simulink model "autosar"  (R2021a)
settings: Solver=FixedStepDiscrete  StartTime=0.0  StopTime=10.0  RelTol=1e-3  EnableMultiTasking=on
libraries: autosarlibdem x1, autosarspkglib_internal x1
settings Model: Creator=Aly  LastModifiedBy=Aly
settings SolverCC: AlgebraicLoopSolver=TrustRegion  AutoInsertRateTranBlk=on  InsertRTBMode=Never (minimum delay)
settings OptimizationCC: DefaultParameterBehavior=Inlined  EnhancedBackFolding=on  PassReuseOutputArgsAs=Individual arguments  ZeroExternalMemoryAtStartup=off  ZeroInternalMemoryAtStartup=off  OptimizeBlockOrder=speed  DifferentSizesBufferReuse=on  OptimizationCustomize=off  EfficientTunableParamExpr=on
settings DebuggingCC: MultiTaskDSMMsg=none  MultiTaskRateTransMsg=warning  ParameterTunabilityLossMsg=error  UnconnectedInputMsg=none  UnconnectedOutputMsg=none  SFMachineParentedDataDiag=warning
settings SFSimCC: MATLABDynamicMemAlloc=off
settings RTWCC: Description=AUTOSAR  SystemTargetFile=autosar.tlc  GenCodeOnly=on  TemplateMakefile=ert_default_tmf  IncludeHyperlinkInReport=on
settings CodeAppCC: ForceParamTrailComments=on  IgnoreCustomStorageClasses=off  OperatorAnnotations=on  SimulinkDataObjDesc=on  SFDataObjDesc=on  InsertBlockDesc=on
settings STFCustomTargetCC: TargetLangStandard=C99 (ISO)  MultiwordLength=256  ParMdlRefBuildCompliant=on  CompOptLevelCompliant=on  IncludeMdlTerminateFcn=off  CombineOutputUpdateFcns=on  SuppressErrorStatus=on  ERTCustomFileBanners=on  SupportNonFinite=off  SupportComplex=off  SupportContinuousTime=off  SupportNonInlinedSFcns=off  RemoveResetFunc=on  MATLABClassNameForMDSCustomization=Simulink.SoftwareTarget.ERTCustomization  AutosarCompliant=on  GRTInterface=off  LookupTableObjectStructAxisOrder=2,1,3,4,...  LUTObjectStructOrderEvenSpacing=Size,Table,Breakpoints  SystemTargetFile=autosar.tlc
settings ERTTargetCC: TargetLangStandard=C99 (ISO)  ConcurrentExecutionCompliant=off  IncludeMdlTerminateFcn=off  SuppressErrorStatus=on  SupportNonFinite=off  SupportComplex=off  ModelStepFunctionPrototypeControlCompliant=off  CPPClassGenCompliant=off  AutosarCompliant=on  LookupTableObjectStructAxisOrder=2,1,3,4,...  LUTObjectStructOrderEvenSpacing=Size,Table,Breakpoints  InlinedParameterPlacement=NonHierarchical  ERTCustomFileTemplate=example_file_process.tlc

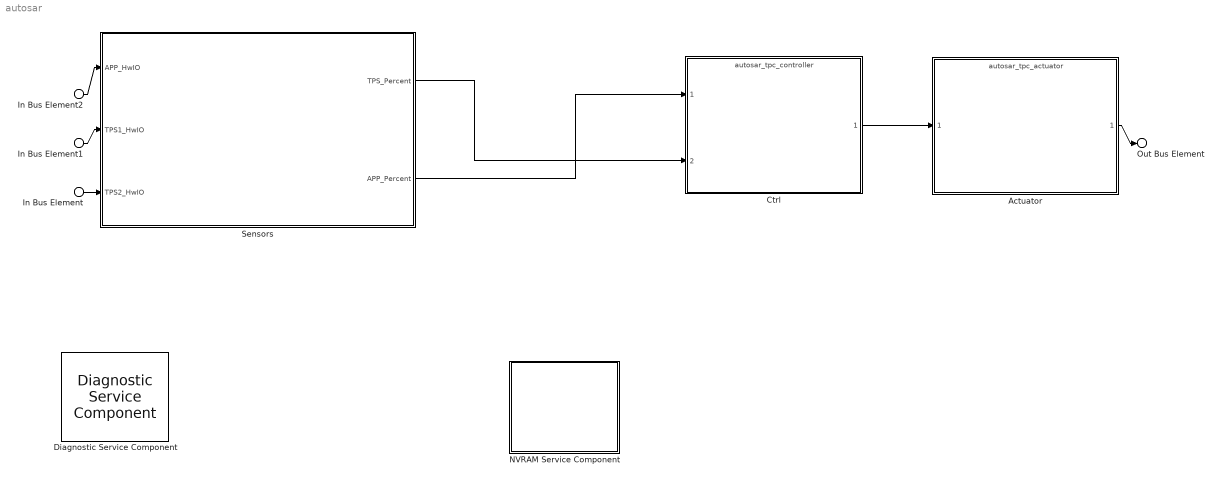
== system autosar ==
  In Bus Element2 : Inport  PortName=APP_HwIO
  In Bus Element1 : Inport  Port=2  PortName=TPS2_HwIO1
  In Bus Element : Inport  Port=3  PortName=TPS1_HwIO
  Actuator : ModelReference  ModelNameDialog=autosar_tpc_actuator  SimulationMode=Normal  ScheduleRates=on  ScheduleRatesWith=Schedule Editor  CodeInterface=Top model  ModelReferenceVersion=3.0
      settings: PortSchema="{\"entries\":[{\"content\":{\"headerSize\":38,\"margin\":15,\"minimumSpacing\":25,\"sides\":[{\"content\":{\"connectorIds\":[\"In1\"]},\"type\":\"ConnectorPlacement.EquallySpacedRectSide\",\"uuid\":\"26fd7ed6-1773-482a-a7b4-c0bab0c01c6e\"},{\"content\":{\"connectorIds\":[\"Out1\"],\"side\":\"RIGHT\"},\"type\":\"ConnectorPlacement.EquallySpacedRectSide\",\"uuid\":\"76751916-8837-4aff-8479-b4617ededb25\"},{\"content\":{\"connectorIds\":[],\"side\":\"TOP\"},\"type\":\"ConnectorPlacement.EquallySpacedRectSide\",\"uuid\":\"b9915de3-15c1-4354-81f8-a4ac649be3ef\"}]},\"type\":\"ConnectorPlacement.EquallySpacedConnector\",\"uuid\":\"5d928bdd-7cbf-4ffd-a89b-6f4194195412\"}],\"packageUris\":[\"http://schema.mathworks.com/mf0/Connector/19700101\"],\"version\":\"1.0\"}"
  Ctrl : ModelReference  ModelNameDialog=autosar_tpc_controller.slx  SimulationMode=Normal  ScheduleRates=on  ScheduleRatesWith=Schedule Editor  ModelReferenceVersion=3.0
      settings: PortSchema="{\"entries\":[{\"content\":{\"headerSize\":38,\"margin\":15,\"minimumSpacing\":25,\"sides\":[{\"content\":{\"connectorIds\":[\"In1\",\"In2\"]},\"type\":\"ConnectorPlacement.EquallySpacedRectSide\",\"uuid\":\"26fd7ed6-1773-482a-a7b4-c0bab0c01c6e\"},{\"content\":{\"connectorIds\":[\"Out1\"],\"side\":\"RIGHT\"},\"type\":\"ConnectorPlacement.EquallySpacedRectSide\",\"uuid\":\"76751916-8837-4aff-8479-b4617ededb25\"},{\"content\":{\"connectorIds\":[],\"side\":\"TOP\"},\"type\":\"ConnectorPlacement.EquallySpacedRectSide\",\"uuid\":\"b9915de3-15c1-4354-81f8-a4ac649be3ef\"}]},\"type\":\"ConnectorPlacement.EquallySpacedConnector\",\"uuid\":\"5d928bdd-7cbf-4ffd-a89b-6f4194195412\"}],\"packageUris\":[\"http://schema.mathworks.com/mf0/Connector/19700101\"],\"version\":\"1.0\"}"
  Diagnostic Service Component : autosarlibdem/Diagnostic Service Component  ClientPortNames={'S1StuckHigh', 'S1StuckLow', 'S2StuckHigh', 'S2StuckLow', 'TPS', 'TPS1StuckHigh', 'TPS1StuckLow', 'TPS2StuckHigh', 'TPS2StuckLow'}  ClientPortPortDefinedArguments={'1', '2', '3', '4', '5', '1', '2', '3', '4'}  MaxEventId=10  MaxFID=10  DemDebounceCounterIncrementStepSize=1  DemDebounceCounterDecrementStepSize=1  DemDebounceCounterFailedThreshold=2  DemDebounceCounterPassedThreshold=-1  InhibitionMatrix=[0 0 0 0 0 0 0 0 0 0 0;0 0 0 0 0 0 0 0 0 0 0;0 0 0 0 0 0 0 0 0 0 0;0 0 0 0 0 0 0 0 0 0 0;0 0 0 0 0 0 0 0 0 0 0;0 0 0 0 0 0 0 0 0 0 0;0 0 0 0 0 0 0 0 0 0 0;0 0 0 0 0 0 0 0 0 0 0;0 0 0 0 0 0 0 0 0 0 0;0 0 0 0 0 0 0 0 0 0 0;0 0 0 0 0 0 0 0 0 0 0]  EnableConditionIndexes=zeros(257,'uint8')  StorageConditionIndexes=zeros(257,'uint8')
      settings: SourceProductBaseCode=AS
  NVRAM Service Component : Subsystem  DialogController=bsw_create_dialog  mask(NVRAM Service Component){ClientPortNames={'S1LowSetPoint', 'S2LowSetPoint'}, ClientPortPortDefinedArguments={'1', '2'}, MaxBlockId=10}
      mask prompts: ClientPortNames "Application port names:"; ClientPortPortDefinedArguments "Port defined arguments:"; MaxBlockId "Max BlockId:"
      mask help: Configure AUTOSAR NVRAM Services and Runtime Environment (RTE) for emulation.
      mask init:
      | autosar.bsw.Dem_defineIntEnumTypes(bdroot(gcb));
      settings: PreCopyFcn=autosar.bsw.ServiceComponent.preCopyCallback(gcb, bdroot);  PortSchema="{\"entries\":[{\"content\":{\"headerSize\":26,\"margin\":15,\"minimumSpacing\":25,\"sides\":[{\"content\":{\"connectorIds\":[]},\"type\":\"ConnectorPlacement.EquallySpacedRectSide\",\"uuid\":\"194fddf8-ae40-4ae3-8397-8b27cef3d678\"},{\"content\":{\"connectorIds\":[],\"side\":\"RIGHT\"},\"type\":\"ConnectorPlacement.EquallySpacedRectSide\",\"uuid\":\"d15cd58e-997f-46ff-b602-45f4e834c83b\"},{\"content\":{\"connectorIds\":[],\"side\":\"TOP\"},\"type\":\"ConnectorPlacement.EquallySpacedRectSide\",\"uuid\":\"279e8bf3-7635-4781-81a2-9c29f80d2e6e\"}]},\"type\":\"ConnectorPlacement.EquallySpacedConnector\",\"uuid\":\"f28a43c0-52f5-4644-acaf-ed8d54afaf9a\"}],\"packageUris\":[\"http://schema.mathworks.com/mf0/Connector/R2020b\"],\"version\":\"1.0\"}"
      mask Help: helpview(fullfile(docroot,'autosar','helptargets.map'),'autosar_memory_service_block');
      mask DialogControl DescGroupVar Prompt: NVRAM Service Component
  Sensors : Subsystem
      settings: PortSchema="{\"entries\":[{\"content\":{\"headerSize\":26,\"margin\":15,\"minimumSpacing\":25,\"sides\":[{\"content\":{\"connectorIds\":[\"In3\",\"In1\",\"In2\"]},\"type\":\"ConnectorPlacement.EquallySpacedRectSide\",\"uuid\":\"26fd7ed6-1773-482a-a7b4-c0bab0c01c6e\"},{\"content\":{\"connectorIds\":[\"Out1\",\"Out2\"],\"side\":\"RIGHT\"},\"type\":\"ConnectorPlacement.EquallySpacedRectSide\",\"uuid\":\"76751916-8837-4aff-8479-b4617ededb25\"},{\"content\":{\"connectorIds\":[],\"side\":\"TOP\"},\"type\":\"ConnectorPlacement.EquallySpacedRectSide\",\"uuid\":\"b9915de3-15c1-4354-81f8-a4ac649be3ef\"}]},\"type\":\"ConnectorPlacement.EquallySpacedConnector\",\"uuid\":\"5d928bdd-7cbf-4ffd-a89b-6f4194195412\"}],\"packageUris\":[\"http://schema.mathworks.com/mf0/Connector/R2020b\"],\"version\":\"1.0\"}"
  Out Bus Element : Outport  PortName=ThrCmd_HwIO
  wires:
  Ctrl/1 -> Actuator/1
  Actuator/1 -> Out Bus Element/1
  Sensors/1(TPS_Percent) -> Ctrl/2
  In Bus Element2/1 -> Sensors/3(APP_HwIO)
  In Bus Element1/1 -> Sensors/1(TPS1_HwIO)
  In Bus Element/1 -> Sensors/2(TPS2_HwIO)
  Sensors/2(APP_Percent) -> Ctrl/1

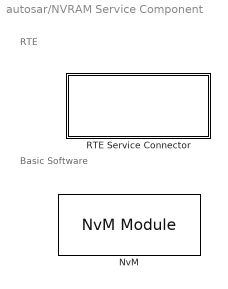
== system autosar/NVRAM Service Component ==
  note: Basic Software
  note: RTE
  NvM : autosarspkglib_internal/NvM Module  MaxBlockId=MaxBlockId
      settings: SourceProductBaseCode=AS
  RTE Service Connector : Subsystem  mask(RTE Service Connector){ApplicationFunctionNames={'S1LowSetPoint_ReadBlock', 'S2LowSetPoint_ReadBlock'}, ServiceFunctionNames={'NvM_ReadBlock', 'NvM_ReadBlock'}, ServicePortDefinedArguments={'1', '2'}}
      mask prompts: ApplicationFunctionNames "Application function names:"; ServiceFunctionNames "Service function names"; ServicePortDefinedArguments "Service port defined arguments:"
      mask help: Connect application callers to service functions.
      settings: PreCopyFcn=autosar.bsw.ServiceComponent.preCopyCallback(gcb, bdroot);  PortSchema="{\"entries\":[{\"content\":{\"headerSize\":26,\"margin\":15,\"minimumSpacing\":25,\"sides\":[{\"content\":{\"connectorIds\":[]},\"type\":\"ConnectorPlacement.EquallySpacedRectSide\",\"uuid\":\"4ecfe5d0-fb5a-48e0-9a95-eb2d0ced430d\"},{\"content\":{\"connectorIds\":[],\"side\":\"RIGHT\"},\"type\":\"ConnectorPlacement.EquallySpacedRectSide\",\"uuid\":\"c9ebb1a9-c36d-4d96-bfa3-5c98d1db5281\"},{\"content\":{\"connectorIds\":[],\"side\":\"TOP\"},\"type\":\"ConnectorPlacement.EquallySpacedRectSide\",\"uuid\":\"1a5cbcf8-dff4-4e62-88af-b7725a5bcda7\"}]},\"type\":\"ConnectorPlacement.EquallySpacedConnector\",\"uuid\":\"7a2d718a-79eb-42fc-b332-1a3d42946146\"}],\"packageUris\":[\"http://schema.mathworks.com/mf0/Connector/R2020b\"],\"version\":\"1.0\"}"
      mask Display: disp(message('autosarstandard:ui:uiRteServiceConnector').getString());

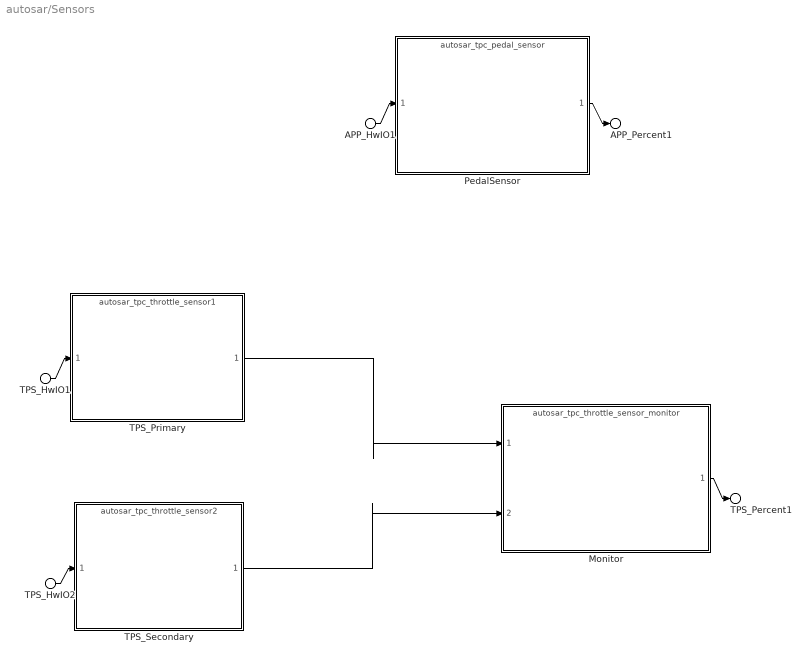
== system autosar/Sensors ==
  TPS_HwIO1 : Inport  PortName=TPS1_HwIO
  TPS_HwIO2 : Inport  Port=2  PortName=TPS2_HwIO
  APP_HwIO1 : Inport  Port=3  PortName=APP_HwIO
  Monitor : ModelReference  ModelNameDialog=autosar_tpc_throttle_sensor_monitor.slx  SimulationMode=Normal  ScheduleRates=on  ScheduleRatesWith=Schedule Editor  ModelReferenceVersion=3.0
      settings: PortSchema="{\"entries\":[{\"content\":{\"headerSize\":38,\"margin\":15,\"minimumSpacing\":25,\"sides\":[{\"content\":{\"connectorIds\":[\"In1\",\"In2\"]},\"type\":\"ConnectorPlacement.EquallySpacedRectSide\",\"uuid\":\"26fd7ed6-1773-482a-a7b4-c0bab0c01c6e\"},{\"content\":{\"connectorIds\":[\"Out1\"],\"side\":\"RIGHT\"},\"type\":\"ConnectorPlacement.EquallySpacedRectSide\",\"uuid\":\"76751916-8837-4aff-8479-b4617ededb25\"},{\"content\":{\"connectorIds\":[],\"side\":\"TOP\"},\"type\":\"ConnectorPlacement.EquallySpacedRectSide\",\"uuid\":\"b9915de3-15c1-4354-81f8-a4ac649be3ef\"}]},\"type\":\"ConnectorPlacement.EquallySpacedConnector\",\"uuid\":\"5d928bdd-7cbf-4ffd-a89b-6f4194195412\"}],\"packageUris\":[\"http://schema.mathworks.com/mf0/Connector/19700101\"],\"version\":\"1.0\"}"
  PedalSensor : ModelReference  ModelNameDialog=autosar_tpc_pedal_sensor.slx  SimulationMode=Normal  ScheduleRates=on  ScheduleRatesWith=Schedule Editor  ModelReferenceVersion=3.0
      settings: PortSchema="{\"entries\":[{\"content\":{\"headerSize\":38,\"margin\":15,\"minimumSpacing\":25,\"sides\":[{\"content\":{\"connectorIds\":[\"In1\"]},\"type\":\"ConnectorPlacement.EquallySpacedRectSide\",\"uuid\":\"26fd7ed6-1773-482a-a7b4-c0bab0c01c6e\"},{\"content\":{\"connectorIds\":[\"Out1\"],\"side\":\"RIGHT\"},\"type\":\"ConnectorPlacement.EquallySpacedRectSide\",\"uuid\":\"76751916-8837-4aff-8479-b4617ededb25\"},{\"content\":{\"connectorIds\":[],\"side\":\"TOP\"},\"type\":\"ConnectorPlacement.EquallySpacedRectSide\",\"uuid\":\"b9915de3-15c1-4354-81f8-a4ac649be3ef\"}]},\"type\":\"ConnectorPlacement.EquallySpacedConnector\",\"uuid\":\"5d928bdd-7cbf-4ffd-a89b-6f4194195412\"}],\"packageUris\":[\"http://schema.mathworks.com/mf0/Connector/19700101\"],\"version\":\"1.0\"}"
  TPS_Primary : ModelReference  ModelNameDialog=autosar_tpc_throttle_sensor1.slx  SimulationMode=Normal  ScheduleRates=on  ScheduleRatesWith=Schedule Editor  ModelReferenceVersion=2.1
      settings: PortSchema="{\"entries\":[{\"content\":{\"headerSize\":38,\"margin\":15,\"minimumSpacing\":25,\"sides\":[{\"content\":{\"connectorIds\":[\"In1\"]},\"type\":\"ConnectorPlacement.EquallySpacedRectSide\",\"uuid\":\"26fd7ed6-1773-482a-a7b4-c0bab0c01c6e\"},{\"content\":{\"connectorIds\":[\"Out1\"],\"side\":\"RIGHT\"},\"type\":\"ConnectorPlacement.EquallySpacedRectSide\",\"uuid\":\"76751916-8837-4aff-8479-b4617ededb25\"},{\"content\":{\"connectorIds\":[],\"side\":\"TOP\"},\"type\":\"ConnectorPlacement.EquallySpacedRectSide\",\"uuid\":\"b9915de3-15c1-4354-81f8-a4ac649be3ef\"}]},\"type\":\"ConnectorPlacement.EquallySpacedConnector\",\"uuid\":\"5d928bdd-7cbf-4ffd-a89b-6f4194195412\"}],\"packageUris\":[\"http://schema.mathworks.com/mf0/Connector/19700101\"],\"version\":\"1.0\"}"
  TPS_Secondary : ModelReference  ModelNameDialog=autosar_tpc_throttle_sensor2.slx  SimulationMode=Normal  ScheduleRates=on  ScheduleRatesWith=Schedule Editor  ModelReferenceVersion=2.0
      settings: PortSchema="{\"entries\":[{\"content\":{\"headerSize\":38,\"margin\":15,\"minimumSpacing\":25,\"sides\":[{\"content\":{\"connectorIds\":[\"In1\"]},\"type\":\"ConnectorPlacement.EquallySpacedRectSide\",\"uuid\":\"26fd7ed6-1773-482a-a7b4-c0bab0c01c6e\"},{\"content\":{\"connectorIds\":[\"Out1\"],\"side\":\"RIGHT\"},\"type\":\"ConnectorPlacement.EquallySpacedRectSide\",\"uuid\":\"76751916-8837-4aff-8479-b4617ededb25\"},{\"content\":{\"connectorIds\":[],\"side\":\"TOP\"},\"type\":\"ConnectorPlacement.EquallySpacedRectSide\",\"uuid\":\"b9915de3-15c1-4354-81f8-a4ac649be3ef\"}]},\"type\":\"ConnectorPlacement.EquallySpacedConnector\",\"uuid\":\"5d928bdd-7cbf-4ffd-a89b-6f4194195412\"}],\"packageUris\":[\"http://schema.mathworks.com/mf0/Connector/19700101\"],\"version\":\"1.0\"}"
  TPS_Percent1 : Outport  PortName=TPS_Percent
  APP_Percent1 : Outport  Port=2  PortName=APP_Percent
  wires:
  TPS_HwIO1/1 -> TPS_Primary/1
  TPS_HwIO2/1 -> TPS_Secondary/1
  Monitor/1 -> TPS_Percent1/1
  TPS_Primary/1 -> Monitor/1
  TPS_Secondary/1 -> Monitor/2
  APP_HwIO1/1 -> PedalSensor/1
  PedalSensor/1 -> APP_Percent1/1

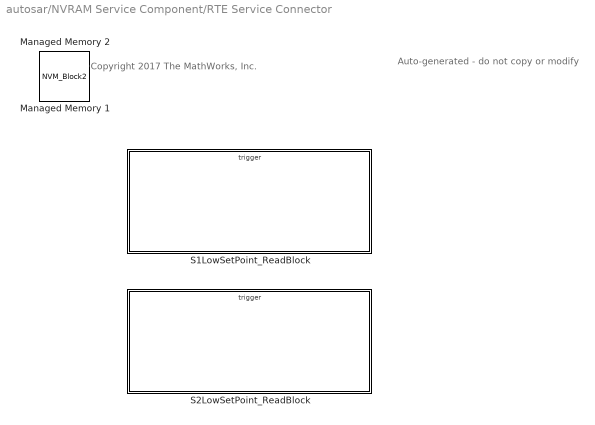
== system autosar/NVRAM Service Component/RTE Service Connector ==
  note: Copyright 2017 The MathWorks, Inc.
  note: Auto-generated - do not copy or modify
  Managed Memory 1 : DataStoreMemory  DataStoreName=NVM_Block1  ShowAdditionalParam=off  OutDataTypeStr=numerictype(0,8,0)  Dimensions=[1;1]
  Managed Memory 2 : DataStoreMemory  DataStoreName=NVM_Block2  ShowAdditionalParam=off  OutDataTypeStr=numerictype(0,8,0)  Dimensions=[1;1]
  S1LowSetPoint_ReadBlock : Subsystem
      settings: PortSchema="{\"entries\":[{\"content\":{\"headerSize\":26,\"margin\":15,\"minimumSpacing\":25,\"sides\":[{\"content\":{\"connectorIds\":[]},\"type\":\"ConnectorPlacement.EquallySpacedRectSide\",\"uuid\":\"5a9da188-ef59-4c66-b468-db01ce971523\"},{\"content\":{\"connectorIds\":[],\"side\":\"RIGHT\"},\"type\":\"ConnectorPlacement.EquallySpacedRectSide\",\"uuid\":\"30a0c68d-457f-49a2-af79-30c22df1fcba\"},{\"content\":{\"connectorIds\":[\"In1\"],\"side\":\"TOP\"},\"type\":\"ConnectorPlacement.EquallySpacedRectSide\",\"uuid\":\"b7342b4d-d64b-4e9b-8740-4f2f54877427\"}]},\"type\":\"ConnectorPlacement.EquallySpacedConnector\",\"uuid\":\"8567af34-33bd-481e-9412-d6ce2e3a6a7a\"}],\"packageUris\":[\"http://schema.mathworks.com/mf0/Connector/R2020b\"],\"version\":\"1.0\"}"
  S2LowSetPoint_ReadBlock : Subsystem
      settings: PortSchema="{\"entries\":[{\"content\":{\"headerSize\":26,\"margin\":15,\"minimumSpacing\":25,\"sides\":[{\"content\":{\"connectorIds\":[]},\"type\":\"ConnectorPlacement.EquallySpacedRectSide\",\"uuid\":\"5a9da188-ef59-4c66-b468-db01ce971523\"},{\"content\":{\"connectorIds\":[],\"side\":\"RIGHT\"},\"type\":\"ConnectorPlacement.EquallySpacedRectSide\",\"uuid\":\"30a0c68d-457f-49a2-af79-30c22df1fcba\"},{\"content\":{\"connectorIds\":[\"In1\"],\"side\":\"TOP\"},\"type\":\"ConnectorPlacement.EquallySpacedRectSide\",\"uuid\":\"b7342b4d-d64b-4e9b-8740-4f2f54877427\"}]},\"type\":\"ConnectorPlacement.EquallySpacedConnector\",\"uuid\":\"8567af34-33bd-481e-9412-d6ce2e3a6a7a\"}],\"packageUris\":[\"http://schema.mathworks.com/mf0/Connector/R2020b\"],\"version\":\"1.0\"}"

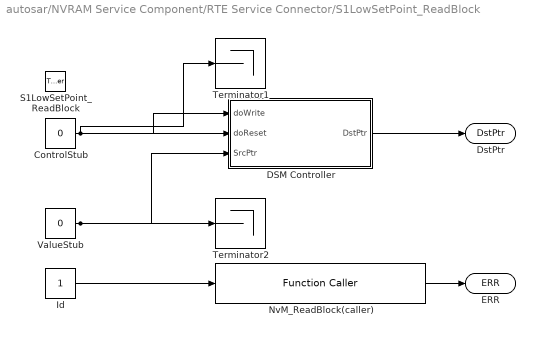
== system autosar/NVRAM Service Component/RTE Service Connector/S1LowSetPoint_ReadBlock ==
  S1LowSetPoint_ReadBlock : TriggerPort  TriggerType=function-call  IsSimulinkFunction=on  FunctionName=S1LowSetPoint_ReadBlock  VariantControl=(inherit)
  ControlStub : Constant  Value=0  OutDataTypeStr=boolean
  DSM Controller : Subsystem  mask(NVRAM DSM Controller){BlockId=1, blockMaskType=numerictype(0,8,0), blockMaskDimensions=[1;1]}
      mask prompts: blockMaskType "Type"; blockMaskDimensions "Dimensions"
      mask help: Used in generated RTE layer to control how NVRAM DSMs are written to and read from.
      mask Callback BlockId:
      | set_param([gcb '/NVRAM_Read'],'DataStoreName',['NVM_Block' num2str(get_param(gcb,'BlockId'))]);
      | set_param([gcb '/NVRAM_Write'],'DataStoreName',['NVM_Block' num2str(get_param(gcb,'BlockId'))]);
      mask Callback blockMaskType:
      | typeStr = get_param(gcb,'blockMaskType');
      | set_param([gcb '/ResetVal'],'OutDataTypeStr',typeStr);
      | defaultVal = autosar.bsw.rte.ManagedDatastoreRTEStrategy.getDefaultTypeStr(typeStr);
      | set_param([gcb '/ResetVal'],'Value',defaultVal);
  Id : Constant  OutDataTypeStr=uint16
  NvM_ReadBlock(caller) : FunctionCaller  FunctionPrototype=ERR = NvM_ReadBlock_ArBlkst(BlockId)
  Terminator1 : Terminator
  Terminator2 : Terminator
  ValueStub : Constant  Value=0  OutDataTypeStr=numerictype(0,8,0)
  DstPtr : ArgOut  OutDataTypeStr=numerictype(0,8,0)  PortDimensions=[1;1]  ArgumentName=DstPtr
  ERR : ArgOut  Port=2  OutDataTypeStr=uint8  ArgumentName=ERR
  wires:
  DSM Controller/1(DstPtr) -> DstPtr/1
  NvM_ReadBlock(caller)/1 -> ERR/1
  ValueStub/1 -> DSM Controller/3(SrcPtr), Terminator2/1
  Id/1 -> NvM_ReadBlock(caller)/1
  ControlStub/1 -> DSM Controller/1(doWrite), DSM Controller/2(doReset), Terminator1/1

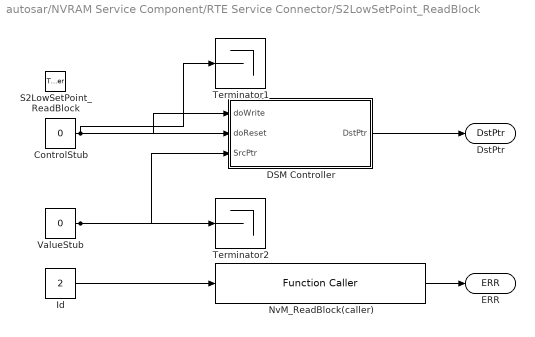
== system autosar/NVRAM Service Component/RTE Service Connector/S2LowSetPoint_ReadBlock ==
  S2LowSetPoint_ReadBlock : TriggerPort  TriggerType=function-call  IsSimulinkFunction=on  FunctionName=S2LowSetPoint_ReadBlock  VariantControl=(inherit)
  ControlStub : Constant  Value=0  OutDataTypeStr=boolean
  DSM Controller : Subsystem  mask(NVRAM DSM Controller){BlockId=2, blockMaskType=numerictype(0,8,0), blockMaskDimensions=[1;1]}
      mask prompts: blockMaskType "Type"; blockMaskDimensions "Dimensions"
      mask help: Used in generated RTE layer to control how NVRAM DSMs are written to and read from.
      mask Callback BlockId:
      | set_param([gcb '/NVRAM_Read'],'DataStoreName',['NVM_Block' num2str(get_param(gcb,'BlockId'))]);
      | set_param([gcb '/NVRAM_Write'],'DataStoreName',['NVM_Block' num2str(get_param(gcb,'BlockId'))]);
      mask Callback blockMaskType:
      | typeStr = get_param(gcb,'blockMaskType');
      | set_param([gcb '/ResetVal'],'OutDataTypeStr',typeStr);
      | defaultVal = autosar.bsw.rte.ManagedDatastoreRTEStrategy.getDefaultTypeStr(typeStr);
      | set_param([gcb '/ResetVal'],'Value',defaultVal);
  Id : Constant  Value=2  OutDataTypeStr=uint16
  NvM_ReadBlock(caller) : FunctionCaller  FunctionPrototype=ERR = NvM_ReadBlock_ArBlkst(BlockId)
  Terminator1 : Terminator
  Terminator2 : Terminator
  ValueStub : Constant  Value=0  OutDataTypeStr=numerictype(0,8,0)
  DstPtr : ArgOut  OutDataTypeStr=numerictype(0,8,0)  PortDimensions=[1;1]  ArgumentName=DstPtr
  ERR : ArgOut  Port=2  OutDataTypeStr=uint8  ArgumentName=ERR
  wires:
  DSM Controller/1(DstPtr) -> DstPtr/1
  NvM_ReadBlock(caller)/1 -> ERR/1
  Id/1 -> NvM_ReadBlock(caller)/1
  ValueStub/1 -> DSM Controller/3(SrcPtr), Terminator2/1
  ControlStub/1 -> DSM Controller/1(doWrite), DSM Controller/2(doReset), Terminator1/1

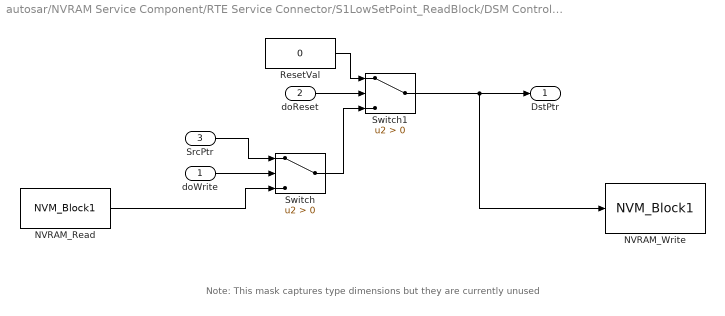
== system autosar/NVRAM Service Component/RTE Service Connector/S1LowSetPoint_ReadBlock/DSM Controller ==
  note: Note: This mask captures type dimensions but they are currently unused
  doWrite : Inport
  doReset : Inport  Port=2
  SrcPtr : Inport  Port=3
  NVRAM_Read : DataStoreRead  Priority=5  DataStoreName=NVM_Block1  IndexOptions=Index vector (dialog)  Indices=1  OutputSizes=1
      settings: AttributesFormatString=Priority: %<Priority>
  NVRAM_Write : DataStoreWrite  DataStoreName=NVM_Block1  IndexOptions=Index vector (dialog)  Indices=1  OutputSizes=1
  ResetVal : Constant  Value=0  OutDataTypeStr=numerictype(0,8,0)
  Switch : Switch  Criteria=u2 > Threshold
  Switch1 : Switch  Criteria=u2 > Threshold
  DstPtr : Outport
  wires:
  ResetVal/1 -> Switch1/1
  NVRAM_Read/1 -> Switch/3
  doWrite/1 -> Switch/2
  Switch/1 -> Switch1/3
  doReset/1 -> Switch1/2
  SrcPtr/1 -> Switch/1
  Switch1/1 -> DstPtr/1, NVRAM_Write/1

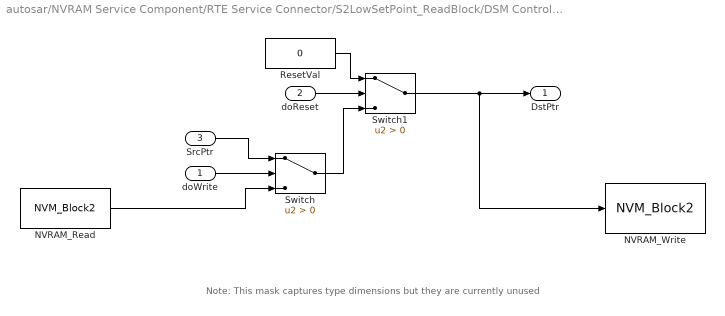
== system autosar/NVRAM Service Component/RTE Service Connector/S2LowSetPoint_ReadBlock/DSM Controller ==
  note: Note: This mask captures type dimensions but they are currently unused
  doWrite : Inport
  doReset : Inport  Port=2
  SrcPtr : Inport  Port=3
  NVRAM_Read : DataStoreRead  Priority=5  DataStoreName=NVM_Block2  IndexOptions=Index vector (dialog)  Indices=1  OutputSizes=1
      settings: AttributesFormatString=Priority: %<Priority>
  NVRAM_Write : DataStoreWrite  DataStoreName=NVM_Block2  IndexOptions=Index vector (dialog)  Indices=1  OutputSizes=1
  ResetVal : Constant  Value=0  OutDataTypeStr=numerictype(0,8,0)
  Switch : Switch  Criteria=u2 > Threshold
  Switch1 : Switch  Criteria=u2 > Threshold
  DstPtr : Outport
  wires:
  ResetVal/1 -> Switch1/1
  NVRAM_Read/1 -> Switch/3
  doWrite/1 -> Switch/2
  Switch/1 -> Switch1/3
  doReset/1 -> Switch1/2
  SrcPtr/1 -> Switch/1
  Switch1/1 -> DstPtr/1, NVRAM_Write/1
